simulink model "Controller_kinematic_bicycle"  (R2018b)
settings: Solver=ode45  StartTime=0.0  StopTime=5  FixedStep=0.002  MaxStep=0.002  RelTol=1e-3
values from neighbouring files (symbols this model uses):
  forward_mode = -1    [main.m]
  K_alpha = 8    [main.m]
  K_beta = -1.5    [main.m]
  K_rho = 3    [main.m]
  L = 2.006    [main.m]
  theta0 = 0    [main.m]
  theta_d = pi/2    (= 1.57079632679)    [main.m]
  x0 = radius * cos((i-1)*pi/4)    [main.m]
  x_d = 0    [main.m]
  y0 = radius * sin((i-1)*pi/4)    [main.m]
  y_d = 0    [main.m]
settings Model: Creator=zhenghe3  LastModifiedBy=zhenghe3
settings SFSimCC: SimUseLocalCustomCode=off
settings RTWCC: RTWUseLocalCustomCode=off

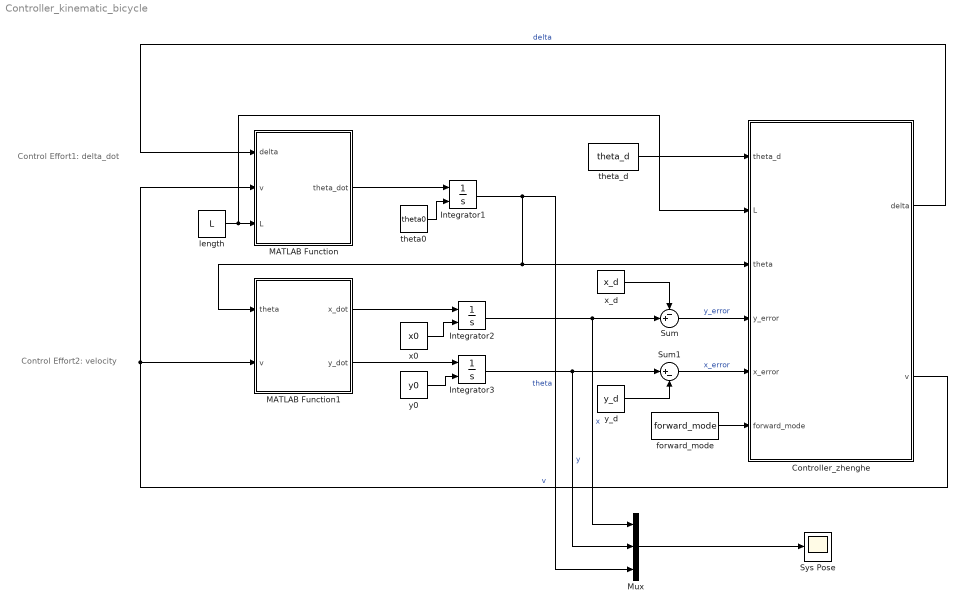
== system Controller_kinematic_bicycle ==
  note: Control Effort2: velocity
  note: Control Effort1: delta_dot
  Controller_zhenghe : Subsystem
  Integrator1 : Integrator  InitialConditionSource=external
  Integrator2 : Integrator  InitialConditionSource=external
  Integrator3 : Integrator  InitialConditionSource=external
  MATLAB Function : MATLAB Function  TreatAsAtomicUnit=on
  MATLAB Function1 : MATLAB Function  TreatAsAtomicUnit=on
  Mux : Mux  Inputs=3
  Sum : Sum  Inputs=-+|
  Sum1 : Sum  Inputs=|+-
  Sys Pose : Scope
  forward_mode : Constant  Value=forward_mode
  length : Constant  Value=L
  theta0 : Constant  Value=theta0
  theta_d : Constant  Value=theta_d
  x0 : Constant  Value=x0
  x_d : Constant  Value=x_d
  y0 : Constant  Value=y0
  y_d : Constant  Value=y_d
  wires:
  Controller_zhenghe/1(delta) -> MATLAB Function/1(delta)  "delta"
  Controller_zhenghe/2(v) -> MATLAB Function/2(v), MATLAB Function1/2(v)  "v"
  length/1 -> Controller_zhenghe/2(L), MATLAB Function/3(L)
  MATLAB Function/1(theta_dot) -> Integrator1/1
  theta0/1 -> Integrator1/2
  Integrator1/1 -> MATLAB Function1/1(theta), Controller_zhenghe/3(theta), Mux/3  "theta"
  x0/1 -> Integrator2/2
  MATLAB Function1/1(x_dot) -> Integrator2/1
  MATLAB Function1/2(y_dot) -> Integrator3/1
  y0/1 -> Integrator3/2
  Integrator2/1 -> Sum/2, Mux/1  "x"
  Integrator3/1 -> Sum1/1, Mux/2  "y"
  x_d/1 -> Sum/1
  y_d/1 -> Sum1/2
  Mux/1 -> Sys Pose/1
  theta_d/1 -> Controller_zhenghe/1(theta_d)
  Sum/1 -> Controller_zhenghe/4(y_error)  "y_error"
  Sum1/1 -> Controller_zhenghe/5(x_error)  "x_error"
  forward_mode/1 -> Controller_zhenghe/6(forward_mode)

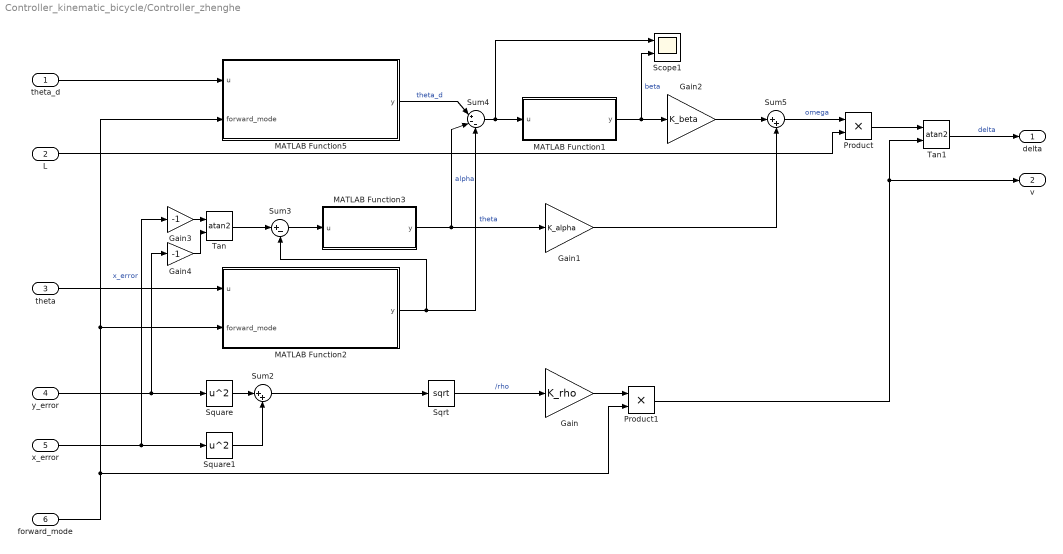
== system Controller_kinematic_bicycle/Controller_zhenghe ==
  theta_d : Inport
  L : Inport  Port=2
  theta : Inport  Port=3
  y_error : Inport  Port=4
  x_error : Inport  Port=5
  forward_mode : Inport  Port=6
  Gain : Gain  Gain=K_rho
  Gain1 : Gain  Gain=K_alpha
  Gain2 : Gain  Gain=K_beta
  Gain3 : Gain  Gain=-1
  Gain4 : Gain  Gain=-1
  MATLAB Function1 : MATLAB Function  TreatAsAtomicUnit=on
  MATLAB Function2 : MATLAB Function  TreatAsAtomicUnit=on
  MATLAB Function3 : MATLAB Function  TreatAsAtomicUnit=on
  MATLAB Function5 : MATLAB Function  TreatAsAtomicUnit=on
  Product : Product
  Product1 : Product
  Scope1 : Scope  NumInputPorts=2
  Sqrt : Sqrt  SaturateOnIntegerOverflow=on
  Square : Math  Operator=square  RndMeth=Zero  SaturateOnIntegerOverflow=on
  Square1 : Math  Operator=square  RndMeth=Zero  SaturateOnIntegerOverflow=on
  Sum2 : Sum  Inputs=|++
  Sum3 : Sum  Inputs=|+-
  Sum4 : Sum  Inputs=|+--
  Sum5 : Sum  Inputs=|++
  Tan : Trigonometry  Operator=atan2
  Tan1 : Trigonometry  Operator=atan2
  delta : Outport
  v : Outport  Port=2
  wires:
  theta_d/1 -> MATLAB Function5/1(u)
  Sum2/1 -> Sqrt/1
  Sum3/1 -> MATLAB Function3/1(u)
  Gain2/1 -> Sum5/1
  Tan/1 -> Sum3/1
  Sum4/1 -> Scope1/1, MATLAB Function1/1(u)
  Product/1 -> Tan1/1
  y_error/1 -> Gain4/1, Square/1
  x_error/1 -> Gain3/1, Square1/1  "x_error"
  Square1/1 -> Sum2/2
  Gain4/1 -> Tan/2
  Square/1 -> Sum2/1
  L/1 -> Product/2
  Sqrt/1 -> Gain/1  "/rho"
  Gain3/1 -> Tan/1
  Gain1/1 -> Sum5/2
  Sum5/1 -> Product/1  "omega"
  theta/1 -> MATLAB Function2/1(u)
  MATLAB Function1/1(y) -> Scope1/2, Gain2/1  "beta"
  forward_mode/1 -> MATLAB Function5/2(forward_mode), MATLAB Function2/2(forward_mode), Product1/2
  Product1/1 -> v/1, Tan1/2
  Gain/1 -> Product1/1
  MATLAB Function5/1(y) -> Sum4/1  "theta_d"
  MATLAB Function3/1(y) -> Sum4/2, Gain1/1  "alpha"
  MATLAB Function2/1(y) -> Sum4/3, Sum3/2  "theta"
  Tan1/1 -> delta/1  "delta"

== matlab function Controller_kinematic_bicycle/MATLAB Function1 ==
  data: theta input; x_dot output; v input; y_dot output
function [x_dot, y_dot] = calc_xy(theta, v)

x_dot = cos(theta) * v;
y_dot = sin(theta) * v;

== matlab function Controller_kinematic_bicycle/MATLAB Function ==
  data: delta input; theta_dot output; v input; L input
function theta_dot = calc_theta_dot(delta, v, L)

theta_dot = v * tan(delta) / L;

== matlab function Controller_kinematic_bicycle/Controller_zhenghe/MATLAB Function2 ==
  data: u input; y output; forward_mode input
function y = calc_real_angle(u, forward_mode)
y = u;

% if the motion should be backward, add a PI to theta
if forward_mode == -1
    y = u + pi;
end

% constrain the output angle into the range (-pi, pi]
while y > pi
    y = y - 2*pi;
end
while y < -pi
    y = y + 2*pi;
end

end

== matlab function Controller_kinematic_bicycle/Controller_zhenghe/MATLAB Function1 ==
  data: u input; y output
function y = calc_real_angle02(u)
y = u;

% constrain the output angle into the range (-pi, pi]
while y > pi
    y = y - 2*pi;
end
while y < -pi
    y = y + 2*pi;
end

end

== matlab function Controller_kinematic_bicycle/Controller_zhenghe/MATLAB Function3 ==
  data: u input; y output
function y = calc_real_angle02(u)
y = u;

% constrain the output angle into the range (-pi, pi]
while y > pi
    y = y - 2*pi;
end
while y < -pi
    y = y + 2*pi;
end

end

== matlab function Controller_kinematic_bicycle/Controller_zhenghe/MATLAB Function5 ==
  data: u input; y output; forward_mode input
function y = calc_real_angle(u, forward_mode)
y = u;

% if the motion should be backward, add a PI to theta
if forward_mode == -1
    y = u + pi;
end

% constrain the output angle into the range (-pi, pi]
while y > pi
    y = y - 2*pi;
end
while y < -pi
    y = y + 2*pi;
end

end
